simulink model "linear_model"  (R2022b)
settings: Solver=VariableStepAuto  StartTime=0.0  StopTime=10  RelTol=1e-3
values from neighbouring files (symbols this model uses):
  A = [-3.78172659857e-08 0 0 0 2.97308e-08 0 0 0 0 1 5.79554624069e-35 6.21514719717e-19 ... (144 elements, 12x12)]    [A1.mat]    (also in A2.mat = [-3.78172659857e-08 0 0 0 2.97308e-08 0 0 0 0 1 -4.775625166; A3.mat = [-3.78172659857e-08 0 0 0 2.97308e-08 0 0 0 0 1 1.7488204834; A4.mat = [-3.78172659857e-08 0 0 0 2.97308e-08 0 0 0 0 1 -4.775625166)
  B = [-5.75123705385 0 0 0 10.0487888864 0 0 0 0 0 0 0 ... (48 elements, 12x4)]    [B1.mat]    (also in B2.mat = [-5.75123707143 0 0 0 10.0487889171 0 0 0 0 0 0 0 ... (48 el; B3.mat = [-5.75123705387 0 0 0 10.0487888865 0 0 0 0 0 0 0 ... (48 el; B4.mat = [-5.75123707143 0 0 0 10.0487889171 0 0 0 0 0 0 0 ... (48 el)
undefined symbols (not defined in the file or in its folder): C, D
settings Model: Creator=henrr  LastModifiedBy=henrr
settings DataIOCC: SaveOutput=off  SaveTime=off  ReturnWorkspaceOutputs=off

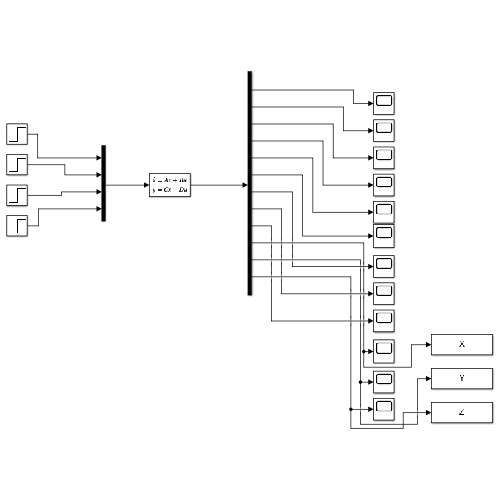
[thumbnail: Simulink's stored preview of the top-level diagram]
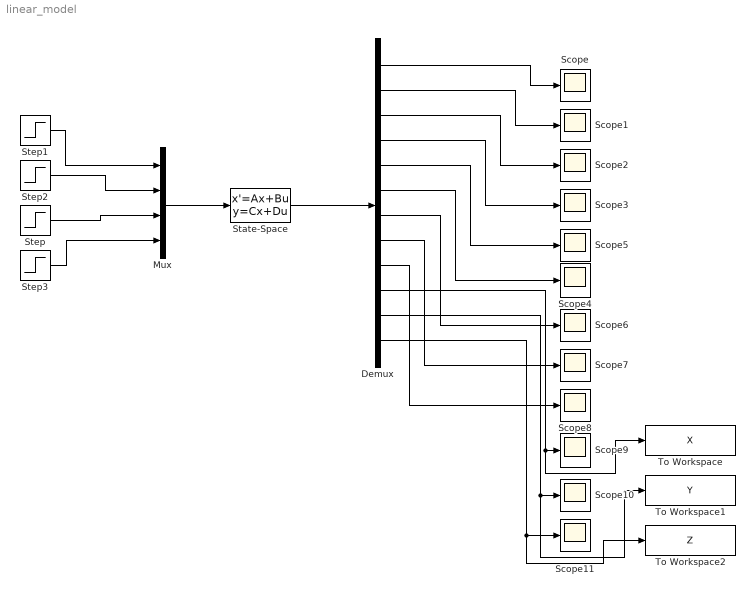
== system linear_model ==
  Demux : Demux  Outputs=12
  Mux : Mux
  Scope{,1..11} (12 alike) : Scope
  State-Space : StateSpace  A=A  B=B  C=C  D=D  InitialCondition=[0 0 0 0 0 0 0 0 0 20 10 20]  AllowTunableDMatrix=on
  Step : Step  Time=0  SampleTime=0
  Step1 : Step  Time=0  After=0  SampleTime=0
  Step2 : Step  Time=0  After=0  SampleTime=0
  Step3 : Step  Time=0  After=0  SampleTime=0
  To Workspace : ToWorkspace  VariableName=X  SaveFormat=Timeseries  SampleTime=-1
  To Workspace1 : ToWorkspace  VariableName=Y  SaveFormat=Timeseries  SampleTime=-1
  To Workspace2 : ToWorkspace  VariableName=Z  SaveFormat=Timeseries  SampleTime=-1
  wires:
  Mux/1 -> State-Space/1
  Step/1 -> Mux/3
  Step1/1 -> Mux/1
  Step2/1 -> Mux/2
  Step3/1 -> Mux/4
  State-Space/1 -> Demux/1
  Demux/3 -> Scope2/1
  Demux/6 -> Scope4/1
  Demux/1 -> Scope/1
  Demux/10 -> To Workspace/1, Scope9/1
  Demux/12 -> To Workspace2/1, Scope11/1
  Demux/11 -> To Workspace1/1, Scope10/1
  Demux/2 -> Scope1/1
  Demux/9 -> Scope8/1
  Demux/4 -> Scope3/1
  Demux/8 -> Scope7/1
  Demux/7 -> Scope6/1
  Demux/5 -> Scope5/1
